simulink model "Block_Diagram_Simulink_2"  (R2023b)
settings: Solver=VariableStepAuto  StartTime=0.0  StopTime=20  RelTol=1e-3
values from neighbouring files (symbols this model uses):
  G1_den = [1 0 0]    [Block_Diagram_2.m]    (also in CSE_Lab3_BlockDiagram1.m)
  G1_num = [1]    [Block_Diagram_2.m]    (also in CSE_Lab3_BlockDiagram1.m = 1)
  G2_den = [1 1]    [Block_Diagram_2.m]    (also in CSE_Lab3_BlockDiagram1.m)
  G2_num = [1]    [Block_Diagram_2.m]    (also in CSE_Lab3_BlockDiagram1.m = 1)
  G3_den = [1 0]    [Block_Diagram_2.m]    (also in CSE_Lab3_BlockDiagram1.m)
  G3_num = [1]    [Block_Diagram_2.m]    (also in CSE_Lab3_BlockDiagram1.m = 1)
  G4_den = [2 0]    [Block_Diagram_2.m]
  G4_num = [1]    [Block_Diagram_2.m]
  H1_den = [1 0]    [Block_Diagram_2.m]    (also in CSE_Lab3_BlockDiagram1.m)
  H1_num = [1]    [Block_Diagram_2.m]    (also in CSE_Lab3_BlockDiagram1.m = 1)
  H2_den = [1 -1]    [Block_Diagram_2.m]    (also in CSE_Lab3_BlockDiagram1.m)
  H2_num = [1]    [Block_Diagram_2.m]    (also in CSE_Lab3_BlockDiagram1.m = 1)
  H3_den = [1 -2]    [Block_Diagram_2.m]    (also in CSE_Lab3_BlockDiagram1.m)
  H3_num = [1]    [Block_Diagram_2.m]    (also in CSE_Lab3_BlockDiagram1.m = 1)
settings Model: Creator=Sofia  LastModifiedBy=Sofia

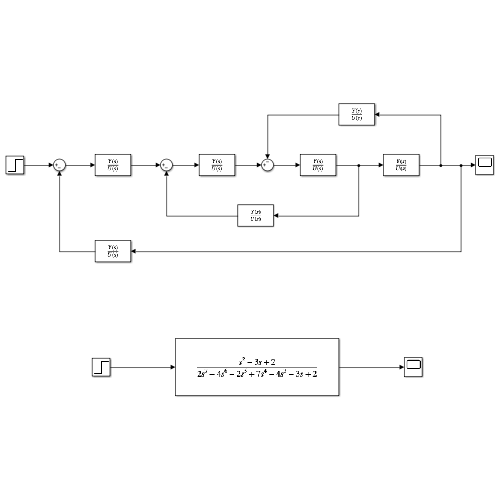
[thumbnail: Simulink's stored preview of the top-level diagram]
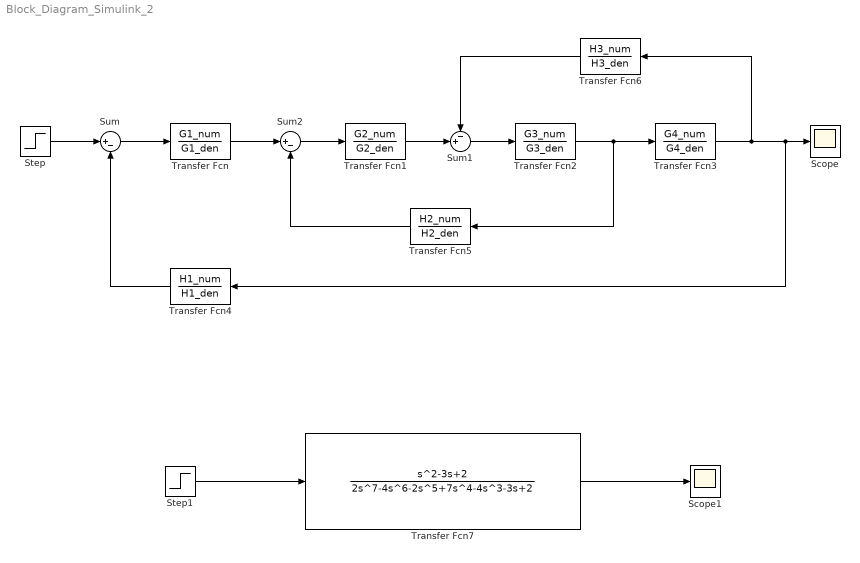
== system Block_Diagram_Simulink_2 ==
  Scope : Scope
  Scope1 : Scope
  Step : Step  Time=0.1  SampleTime=0
  Step1 : Step  SampleTime=0
  Sum : Sum  Inputs=|+-
  Sum1 : Sum  Inputs=-+|
  Sum2 : Sum  Inputs=|+-
  Transfer Fcn : TransferFcn  Numerator=G1_num  Denominator=G1_den
  Transfer Fcn1 : TransferFcn  Numerator=G2_num  Denominator=G2_den
  Transfer Fcn2 : TransferFcn  Numerator=G3_num  Denominator=G3_den
  Transfer Fcn3 : TransferFcn  Numerator=G4_num  Denominator=G4_den
  Transfer Fcn4 : TransferFcn  Numerator=H1_num  Denominator=H1_den
  Transfer Fcn5 : TransferFcn  Numerator=H2_num  Denominator=H2_den
  Transfer Fcn6 : TransferFcn  Numerator=H3_num  Denominator=H3_den
  Transfer Fcn7 : TransferFcn  Numerator=[1 -3 2]  Denominator=[2 -4 -2 7 -4 0 -3 2]
  wires:
  Step/1 -> Sum/1
  Sum/1 -> Transfer Fcn/1
  Transfer Fcn/1 -> Sum2/1
  Sum2/1 -> Transfer Fcn1/1
  Transfer Fcn1/1 -> Sum1/2
  Sum1/1 -> Transfer Fcn2/1
  Transfer Fcn2/1 -> Transfer Fcn5/1, Transfer Fcn3/1
  Transfer Fcn3/1 -> Transfer Fcn6/1, Transfer Fcn4/1, Scope/1
  Transfer Fcn4/1 -> Sum/2
  Transfer Fcn5/1 -> Sum2/2
  Transfer Fcn6/1 -> Sum1/1
  Step1/1 -> Transfer Fcn7/1
  Transfer Fcn7/1 -> Scope1/1
